simulink model "SAT_UNS"  (Simulink 3.00)
settings: Solver=ode45  SolverMode=SingleTasking  StartTime=0.0  StopTime=100  MaxStep=0.10  RelTol=1e-3  AbsTol=1e-3
undefined symbols (not defined in the file or in its folder): sat
settings Model: TimeSaveName=t  SaveOutput=off

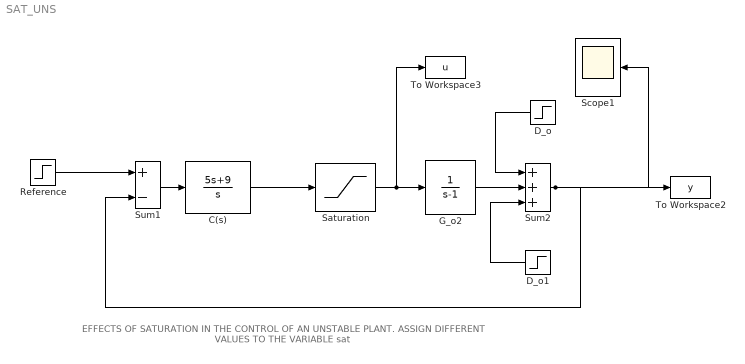
== system SAT_UNS ==
  note: EFFECTS OF SATURATION IN THE CONTROL OF AN UNSTABLE PLANT.
      | ASSIGN DIFFERENT VALUES TO THE VARIABLE sat
  C(s) : TransferFcn  Numerator=[5 9]  Denominator=[1 0]
  D_o : Step  Orientation=left  Time=10  Before=0  After=-0.8  SampleTime=0
  D_o1 : Step  Orientation=left  Time=10.5  Before=0  After=0.8  SampleTime=0
  G_o2 : TransferFcn  Numerator=1  Denominator=[1 -1]
  Reference : Step  Time=1  Before=0  After=1  SampleTime=0
  Saturation : Saturate  UpperLimit=sat  LowerLimit=-sat
  Scope1 : Scope
      settings: TickLabels=on  TimeRange=100.000000  YMin=-4  YMax=4  SaveToWorkspace=off  SaveName=ScopeData  DataFormat=Matrix
  Sum1 : Sum  Inputs=+-  SaturateOnIntegerOverflow=on
  Sum2 : Sum  Inputs=+++  SaturateOnIntegerOverflow=on
  To Workspace2 : ToWorkspace  VariableName=y  SampleTime=0  SaveFormat=Matrix
      settings: Buffer=10000
  To Workspace3 : ToWorkspace  VariableName=u  SampleTime=0  SaveFormat=Matrix
      settings: Buffer=10000
  wires:
  Sum1/1 -> C(s)/1
  C(s)/1 -> Saturation/1
  Saturation/1 -> G_o2/1, To Workspace3/1
  G_o2/1 -> Sum2/2
  Sum2/1 -> To Workspace2/1, Sum1/2, Scope1/1
  D_o/1 -> Sum2/1
  D_o1/1 -> Sum2/3
  Reference/1 -> Sum1/1
